simulink model "m02"  (R2023b)
settings: Solver=VariableStepAuto  StartTime=0.0  StopTime=0.1  RelTol=1e-3
settings Model: Creator=asus  LastModifiedBy=asus

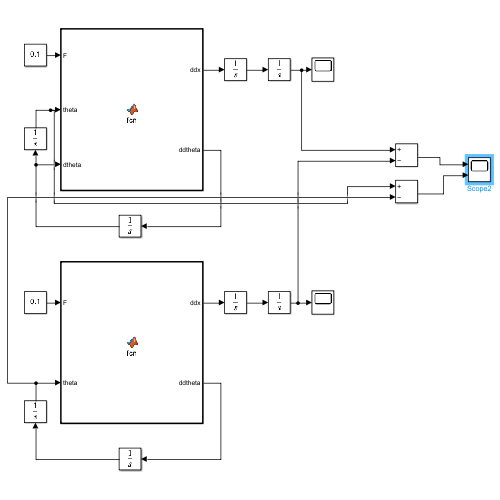
[thumbnail: Simulink's stored preview of the top-level diagram]
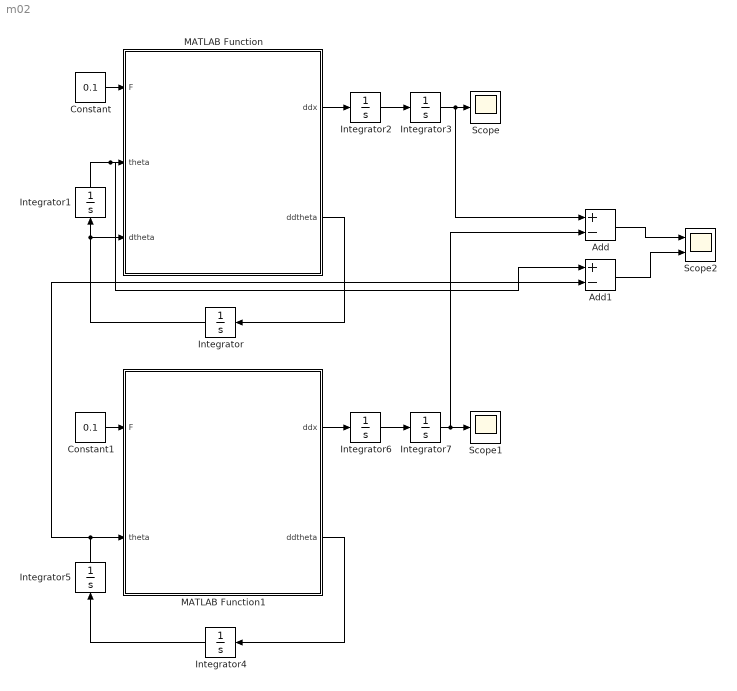
== system m02 ==
  Add : Sum  Inputs=+-
  Add1 : Sum  Inputs=+-
  Constant : Constant  Value=0.1
  Constant1 : Constant  Value=0.1
  Integrator{,1..7} (8 alike) : Integrator
  MATLAB Function : MATLAB Function  TreatAsAtomicUnit=on
  MATLAB Function1 : MATLAB Function  TreatAsAtomicUnit=on
  Scope : Scope
  Scope1 : Scope
  Scope2 : Scope  NumInputPorts=2
  wires:
  Constant/1 -> MATLAB Function/1(F)
  MATLAB Function/2(ddtheta) -> Integrator/1
  Integrator/1 -> MATLAB Function/3(dtheta), Integrator1/1
  Integrator1/1 -> Add1/1, MATLAB Function/2(theta)
  MATLAB Function/1(ddx) -> Integrator2/1
  Integrator2/1 -> Integrator3/1
  Integrator3/1 -> Add/1, Scope/1
  Integrator7/1 -> Add/2, Scope1/1
  Integrator6/1 -> Integrator7/1
  MATLAB Function1/1(ddx) -> Integrator6/1
  Integrator5/1 -> MATLAB Function1/2(theta), Add1/2
  Integrator4/1 -> Integrator5/1
  MATLAB Function1/2(ddtheta) -> Integrator4/1
  Constant1/1 -> MATLAB Function1/1(F)
  Add/1 -> Scope2/1
  Add1/1 -> Scope2/2

== matlab function m02/MATLAB Function1 ==
  data: F input; ddx output; theta input; ddtheta output
function [ddx,ddtheta] = fcn(F,theta)

ddx = -6*theta + 0.8*F;
ddtheta = 40*theta-2.0*F;

== matlab function m02/MATLAB Function ==
  data: F input; ddx output; theta input; dtheta input; ddtheta output
function [ddx,ddtheta] = fcn(F,theta,dtheta)

ddx = 0.12*F + 0.036*sin(theta)*dtheta^2 - 0.9*sin(theta)*cos(theta);
ddx = ddx / ( 0.24 - 0.09*cos(theta)^2 );

ddtheta = 0.3*cos(theta)*F + 0.09*sin(theta)*cos(theta)*dtheta^2 - 6*sin(theta);
ddtheta = ddtheta / ( -0.24 + 0.09*cos(theta)^2 );
